simulink model "stabilita_1"  (R2018a)
settings: Solver=VariableStepAuto  StartTime=0.0  StopTime=100  RelTol=1e-3
undefined symbols (not defined in the file): x10, x20
libraries: simulink x1
settings Model: Creator=vejvarm  LastModifiedBy=vejvarm

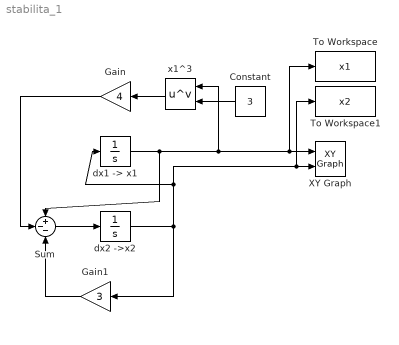
== system stabilita_1 ==
  Constant : Constant  Value=3
  Gain : Gain  Gain=4
  Gain1 : Gain  Gain=3
  Sum : Sum  Inputs=+--
  To Workspace : ToWorkspace  VariableName=x1  SaveFormat=Timeseries  SampleTime=-1
  To Workspace1 : ToWorkspace  VariableName=x2  SaveFormat=Timeseries  SampleTime=-1
  XY Graph : simulink/Sinks/XY Graph  xmin=-5  xmax=5  ymin=-5  ymax=5  st=-1
  "dx1 -> x1" : Integrator  InitialCondition=x10
  dx2 ->x2 : Integrator  InitialCondition=x20
  x1^3 : Math  Operator=pow  RndMeth=Zero  SaturateOnIntegerOverflow=on
  wires:
  Sum/1 -> dx2 ->x2/1
  "dx1 -> x1"/1 -> Sum/1, x1^3/1, To Workspace/1, XY Graph/1
  x1^3/1 -> Gain/1
  Gain/1 -> Sum/2
  dx2 ->x2/1 -> Gain1/1, To Workspace1/1, XY Graph/2, "dx1 -> x1"/1
  Gain1/1 -> Sum/3
  Constant/1 -> x1^3/2
